simulink model "MUSIC_repo_DA_I"  (R2016a)
settings: Solver=VariableStepAuto  StartTime=0.0  StopTime=20000  RelTol=1e-3
undefined symbols (not defined in the file): S_V
libraries: xbsIndex_r4 x785, hdlsllib x7, dspbuff3 x7, dspswit3 x1
(part 1 of 8)
settings Model: Creator=Test  LastModifiedBy=Home

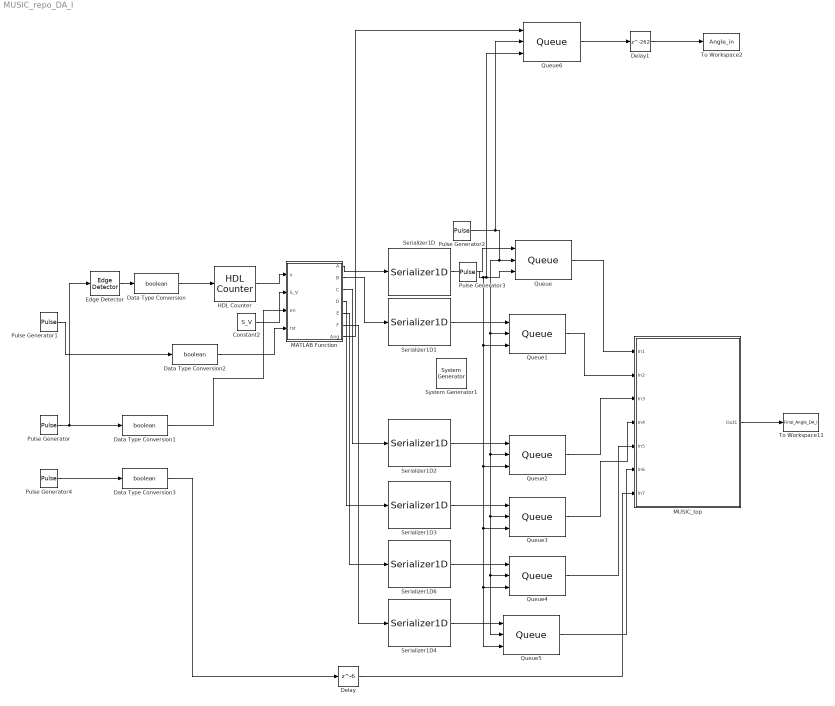
== system MUSIC_repo_DA_I ==
  " System Generator1" : xbsIndex_r4/ System Generator  Tag=genX  xilinxfamily=zynq  part=xc7z020  speed=-1  package=clg484  synthesis_tool=Vivado  clock_wrapper=Clock Enables  directory=C:/Users/Home/Desktop/Patent/Response_to_reviews_25_Feb/MUSIC_nopt  proj_type=Vivado  Synth_file=Vivado Synthesis Defaults  Impl_file=Vivado Implementation Defaults  testbench=on  simulink_period=1  sysclk_period=10  dcm_input_clock_period=10  incr_netlist=off  trim_vbits=Everywhere in SubSystem  dbl_ovrd=According to Block Masks  core_generation=According to Block Masks  run_coregen=off  deprecated_control=off  eval_field=0  block_type=sysgen
  Constant2 : Constant  Value=S_V
  Data Type Conversion{,1..3} (4 alike) : DataTypeConversion  OutDataTypeStr=boolean
  Delay : Delay  DelayLength=6  InitialCondition=0
  Delay1 : Delay  DelayLength=262  InitialCondition=0
  Edge Detector : dspswit3/Edge Detector  InputProcessing=Columns as channels (frame based)
  HDL Counter : hdlsllib/HDL Operations/HDL Counter  CountType=Count limited  CountInit=38  CountStep=1  CountMax=94  CountFromType=Initial value  CountFrom=38  CountResetPort=off  CountLoadPort=off  CountEnbPort=on  CountDirPort=off  CountDataType=Unsigned  CountWordLen=8  CountFracLen=0  CountSampTime=1
  MATLAB Function : MATLAB Function  TreatAsAtomicUnit=on
  MUSIC_top : Subsystem
  Pulse Generator : DiscretePulseGenerator  Period=90  PulseWidth=4  PhaseDelay=2
  Pulse Generator1 : DiscretePulseGenerator  Period=360
  Pulse Generator2 : DiscretePulseGenerator  PulseType=Time based  Period=0.25  PulseWidth=50
  Pulse Generator3 : DiscretePulseGenerator  PulseType=Time based  Period=1  PulseWidth=50
  Pulse Generator4 : DiscretePulseGenerator  Period=352  PulseWidth=4  PhaseDelay=2
  Queue{,1..6} (7 alike) : dspbuff3/Queue  depth=8  trigger=Rising edge  overflow=Dynamic reallocation  pes=Warning  eso=off  fso=off  nso=off  clr=off  clrOutport=off  adf=on
  Serializer1D{,1..4,6} (6 alike) : hdlsllib/HDL Operations/Serializer1D  Ratio=4  IdleCycles=0  validIn=off  startOut=off  validOut=off  inputDataDimensions=-1  inputSampleTime=-1  inputSignalType=auto
  To Workspace11 : ToWorkspace  VariableName=Final_Angle_DA_I  SampleTime=-1
  To Workspace2 : ToWorkspace  VariableName=Angle_in  SampleTime=-1
  wires:
  Data Type Conversion/1 -> HDL Counter/1
  Constant2/1 -> MATLAB Function/2(S_V)
  HDL Counter/1 -> MATLAB Function/1(x)
  Edge Detector/1 -> Data Type Conversion/1
  Pulse Generator1/1 -> Data Type Conversion2/1
  Data Type Conversion2/1 -> MATLAB Function/4(rst)
  Data Type Conversion1/1 -> MATLAB Function/3(en)
  Pulse Generator/1 -> Edge Detector/1, Data Type Conversion1/1
  MATLAB Function/1(A) -> Serializer1D/1
  Serializer1D/1 -> Queue/1
  Pulse Generator4/1 -> Data Type Conversion3/1
  Data Type Conversion3/1 -> Delay/1
  MATLAB Function/2(B) -> Serializer1D1/1
  MATLAB Function/3(C) -> Serializer1D2/1
  MATLAB Function/4(D) -> Serializer1D3/1
  MATLAB Function/5(E) -> Serializer1D6/1
  MATLAB Function/6(F) -> Serializer1D4/1
  Serializer1D1/1 -> Queue1/1
  Serializer1D2/1 -> Queue2/1
  Serializer1D3/1 -> Queue3/1
  Serializer1D6/1 -> Queue4/1
  Serializer1D4/1 -> Queue5/1
  Queue/1 -> MUSIC_top/1(In1)
  Queue1/1 -> MUSIC_top/2(In2)
  Queue2/1 -> MUSIC_top/3(In3)
  Queue3/1 -> MUSIC_top/4(In4)
  Queue4/1 -> MUSIC_top/5(In5)
  Queue5/1 -> MUSIC_top/6(In6)
  Delay/1 -> MUSIC_top/7(In7)
  MUSIC_top/1(Out1) -> To Workspace11/1
  Pulse Generator2/1 -> Queue6/2, Queue/2, Queue2/2, Queue3/2, Queue4/2, Queue5/2, Queue1/2
  Pulse Generator3/1 -> Queue6/3, Queue/3, Queue1/3, Queue2/3, Queue3/3, Queue4/3, Queue5/3
  Queue6/1 -> Delay1/1
  MATLAB Function/7(Ang) -> Queue6/1
  Delay1/1 -> To Workspace2/1

== system MUSIC_repo_DA_I/MUSIC_top ==
  In1 : Inport
  In2 : Inport  Port=2
  In3 : Inport  Port=3
  In4 : Inport  Port=4
  In5 : Inport  Port=5
  In6 : Inport  Port=6
  In7 : Inport  Port=7
  " System Generator1" : xbsIndex_r4/ System Generator  Tag=genX  xilinxfamily=zynq  part=xc7z020  speed=-1  package=clg484  synthesis_tool=Vivado  clock_wrapper=Clock Enables  directory=./res_60  proj_type=Vivado  Synth_file=Vivado Synthesis Defaults  Impl_file=Vivado Implementation Defaults  testbench=off  simulink_period=1  sysclk_period=10  dcm_input_clock_period=10  incr_netlist=off  trim_vbits=Everywhere in SubSystem  dbl_ovrd=According to Block Masks  core_generation=According to Block Masks  run_coregen=off  deprecated_control=off  eval_field=0  block_type=sysgen
  A : xbsIndex_r4/Gateway In  gui_display_data_type=Fixed-point  arith_type=Unsigned  n_bits=14  bin_pt=0  preci_type=Single  exp_width=8  frac_width=24  rows=1  columns=1  quantization="Round  (unbiased: +/- Inf)"  overflow=Saturate  period=1  UseAsADC=off  ADCChannel='1'  interface=None  automatic_assignment=on  address_offset=hex2dec('00')  intf_name=''  intf_description=''  default_value=0  timing_constraint=None  locs_specified=off  LOCs={}  io_standard={}  inherit_from_input=off  hdl_port=on  dbl_ovrd=off  block_type=gatewayin
  B : xbsIndex_r4/Gateway In  gui_display_data_type=Fixed-point  arith_type=Unsigned  n_bits=14  bin_pt=0  preci_type=Single  exp_width=8  frac_width=24  rows=1  columns=1  quantization="Round  (unbiased: +/- Inf)"  overflow=Saturate  period=1  UseAsADC=off  ADCChannel='1'  interface=None  automatic_assignment=on  address_offset=hex2dec('00')  intf_name=''  intf_description=''  default_value=0  timing_constraint=None  locs_specified=off  LOCs={}  io_standard={}  inherit_from_input=off  hdl_port=on  dbl_ovrd=off  block_type=gatewayin
  C : xbsIndex_r4/Gateway In  gui_display_data_type=Fixed-point  arith_type=Unsigned  n_bits=14  bin_pt=0  preci_type=Single  exp_width=8  frac_width=24  rows=1  columns=1  quantization="Round  (unbiased: +/- Inf)"  overflow=Saturate  period=1  UseAsADC=off  ADCChannel='1'  interface=None  automatic_assignment=on  address_offset=hex2dec('00')  intf_name=''  intf_description=''  default_value=0  timing_constraint=None  locs_specified=off  LOCs={}  io_standard={}  inherit_from_input=off  hdl_port=on  dbl_ovrd=off  block_type=gatewayin
  D : xbsIndex_r4/Gateway In  gui_display_data_type=Fixed-point  arith_type=Unsigned  n_bits=14  bin_pt=0  preci_type=Single  exp_width=8  frac_width=24  rows=1  columns=1  quantization="Round  (unbiased: +/- Inf)"  overflow=Saturate  period=1  UseAsADC=off  ADCChannel='1'  interface=None  automatic_assignment=on  address_offset=hex2dec('00')  intf_name=''  intf_description=''  default_value=0  timing_constraint=None  locs_specified=off  LOCs={}  io_standard={}  inherit_from_input=off  hdl_port=on  dbl_ovrd=off  block_type=gatewayin
  E : xbsIndex_r4/Gateway In  gui_display_data_type=Fixed-point  arith_type=Unsigned  n_bits=14  bin_pt=0  preci_type=Single  exp_width=8  frac_width=24  rows=1  columns=1  quantization="Round  (unbiased: +/- Inf)"  overflow=Saturate  period=1  UseAsADC=off  ADCChannel='1'  interface=None  automatic_assignment=on  address_offset=hex2dec('00')  intf_name=''  intf_description=''  default_value=0  timing_constraint=None  locs_specified=off  LOCs={}  io_standard={}  inherit_from_input=off  hdl_port=on  dbl_ovrd=off  block_type=gatewayin
  Enable : xbsIndex_r4/Gateway In  gui_display_data_type=Boolean  arith_type=Boolean  n_bits=14  bin_pt=0  preci_type=Single  exp_width=8  frac_width=24  rows=1  columns=1  quantization="Round  (unbiased: +/- Inf)"  overflow=Saturate  period=1  UseAsADC=off  ADCChannel='1'  interface=None  automatic_assignment=on  address_offset=hex2dec('00')  intf_name=''  intf_description=''  default_value=0  timing_constraint=None  locs_specified=off  LOCs={}  io_standard={}  inherit_from_input=off  hdl_port=on  dbl_ovrd=off  block_type=gatewayin
  F : xbsIndex_r4/Gateway In  gui_display_data_type=Fixed-point  arith_type=Unsigned  n_bits=14  bin_pt=0  preci_type=Single  exp_width=8  frac_width=24  rows=1  columns=1  quantization="Round  (unbiased: +/- Inf)"  overflow=Saturate  period=1  UseAsADC=off  ADCChannel='1'  interface=None  automatic_assignment=on  address_offset=hex2dec('00')  intf_name=''  intf_description=''  default_value=0  timing_constraint=None  locs_specified=off  LOCs={}  io_standard={}  inherit_from_input=off  hdl_port=on  dbl_ovrd=off  block_type=gatewayin
  Final_Angle_DA_I : xbsIndex_r4/Gateway Out  inherit_from_input=off  hdl_port=on  rows=1  columns=1  UseAsDAC=off  DACChannel='1'  interface=None  automatic_assignment=on  address_offset=hex2dec('00')  intf_name=''  intf_description=''  timing_constraint=None  locs_specified=off  LOCs={}  io_standard={}  block_type=gatewayout
  MUSIC : Subsystem
  Out1 : Outport
  wires:
  A/1 -> MUSIC/1(A)
  B/1 -> MUSIC/2(B)
  C/1 -> MUSIC/3(C)
  E/1 -> MUSIC/5(E)
  Enable/1 -> MUSIC/7(EN)
  MUSIC/1(Angle) -> Final_Angle_DA_I/1
  F/1 -> MUSIC/6(F)
  D/1 -> MUSIC/4(D)
  In7/1 -> Enable/1
  In1/1 -> A/1
  In2/1 -> B/1
  In4/1 -> D/1
  In3/1 -> C/1
  In6/1 -> F/1
  In5/1 -> E/1
  Final_Angle_DA_I/1 -> Out1/1

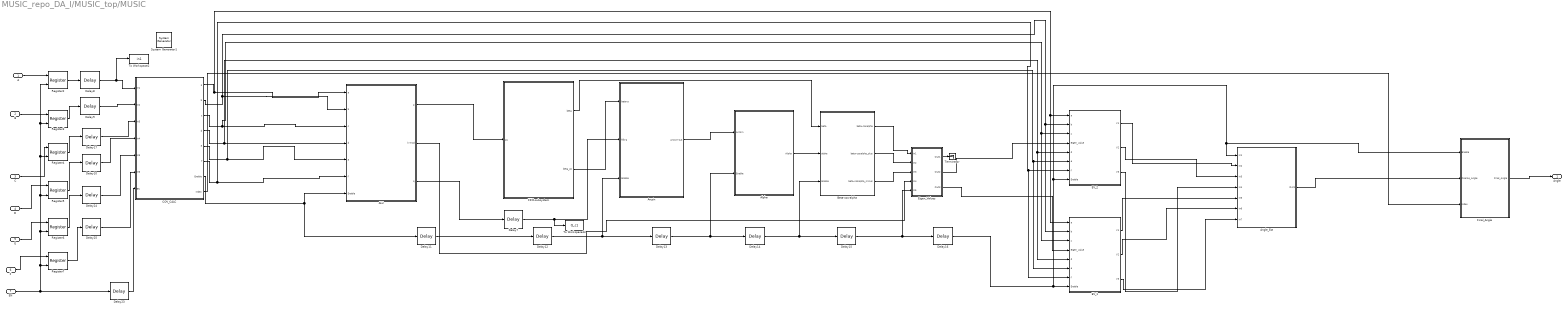
== system MUSIC_repo_DA_I/MUSIC_top/MUSIC ==
  A : Inport
  B : Inport  Port=2
  C : Inport  Port=3
  D : Inport  Port=4
  E : Inport  Port=5
  F : Inport  Port=6
  EN : Inport  Port=7
  " System Generator1" : xbsIndex_r4/ System Generator  Tag=genX  xilinxfamily=zynq  part=xc7z020  speed=-1  package=clg484  synthesis_tool=Vivado  clock_wrapper=Clock Enables  directory=./res_60  proj_type=Vivado  Synth_file=Vivado Synthesis Defaults  Impl_file=Vivado Implementation Defaults  testbench=off  simulink_period=1  sysclk_period=10  dcm_input_clock_period=10  incr_netlist=off  trim_vbits=Everywhere in SubSystem  dbl_ovrd=According to Block Masks  core_generation=According to Block Masks  run_coregen=off  deprecated_control=off  eval_field=0  block_type=sysgen
  ALU : Subsystem
  Alpha : Subsystem
  "Angle_Est " : Subsystem
  Arcsin : Subsystem
  Beta-cos-alpha : Subsystem
  COV_CALC : Subsystem
  Delay{8..10,17,23..25} (7 alike) : xbsIndex_r4/Delay  rst=off  infoeditControl=Selection of Reset will increase slice count due to use of real FFs and instead of SRLs  en=off  latency=9  reg_retiming=off  dbl_ovrd=off  block_type=delay
  Delay11 : xbsIndex_r4/Delay  rst=off  infoeditControl=Selection of Reset will increase slice count due to use of real FFs and instead of SRLs  en=off  latency=15  reg_retiming=off  dbl_ovrd=off  block_type=delay
  Delay12 : xbsIndex_r4/Delay  rst=off  infoeditControl=Selection of Reset will increase slice count due to use of real FFs and instead of SRLs  en=off  latency=10  reg_retiming=off  dbl_ovrd=off  block_type=delay
  Delay13 : xbsIndex_r4/Delay  rst=off  infoeditControl=Selection of Reset will increase slice count due to use of real FFs and instead of SRLs  en=off  latency=56  reg_retiming=off  dbl_ovrd=off  block_type=delay
  Delay14 : xbsIndex_r4/Delay  rst=off  infoeditControl=Selection of Reset will increase slice count due to use of real FFs and instead of SRLs  en=off  latency=2  reg_retiming=off  dbl_ovrd=off  block_type=delay
  Delay15 : xbsIndex_r4/Delay  rst=off  infoeditControl=Selection of Reset will increase slice count due to use of real FFs and instead of SRLs  en=off  latency=13  reg_retiming=off  dbl_ovrd=off  block_type=delay
  Delay16 : xbsIndex_r4/Delay  rst=off  infoeditControl=Selection of Reset will increase slice count due to use of real FFs and instead of SRLs  en=off  latency=1  reg_retiming=off  dbl_ovrd=off  block_type=delay
  Delay7 : xbsIndex_r4/Delay  rst=off  infoeditControl=Selection of Reset will increase slice count due to use of real FFs and instead of SRLs  en=off  latency=11  reg_retiming=off  dbl_ovrd=off  block_type=delay
  EV_1 : Subsystem
  EV_2 : Subsystem
  Eigen_Values : Subsystem
  FIFO-subsystem : Subsystem
  Final_Angle : Subsystem
  Register{2..7} (6 alike) : xbsIndex_r4/Register  init=0  rst=off  en=on  dbl_ovrd=off  block_type=register
  Terminator : Terminator
  To Workspace2 : ToWorkspace  VariableName=in1  SaveFormat=Timeseries  SampleTime=-1
  To Workspace43 : ToWorkspace  VariableName=Q_c1  SaveFormat=Timeseries  SampleTime=-1
  Angle : Outport
  wires:
  Delay13/1 -> Alpha/2(Enable), Delay14/1
  Delay14/1 -> Beta-cos-alpha/3(Enable), Delay15/1
  FIFO-subsystem/1(beta) -> Beta-cos-alpha/1(beta)
  Delay15/1 -> Eigen_Values/5(In5), Delay16/1
  Delay12/1 -> Arcsin/3(Enable), Delay13/1
  ALU/1(p) -> FIFO-subsystem/1(p1)
  Delay11/1 -> Delay12/1
  EV_2/3(V3) -> "Angle_Est "/4(In4)
  EV_1/3(V3) -> "Angle_Est "/7(In7)
  A/1 -> Register2/1
  Delay16/1 -> EV_1/8(Enable), EV_2/8(Enable), Final_Angle/1(Enable), "Angle_Est "/1(In1)
  EV_2/1(V1) -> "Angle_Est "/2(In2)
  EV_2/2(V2) -> "Angle_Est "/3(In3)
  EN/1 -> Register7/2, Register6/2, Register5/2, Register3/2, Register2/2, Register4/2, Delay23/1
  EV_1/2(V2) -> "Angle_Est "/6(In6)
  EV_1/1(V1) -> "Angle_Est "/5(In5)
  Register2/1 -> Delay8/1
  COV_CALC/2(b) -> EV_2/2(b), EV_1/2(b), ALU/2(b)
  Register6/1 -> Delay24/1
  COV_CALC/3(c) -> ALU/3(c), EV_2/3(c), EV_1/3(c)
  D/1 -> Register5/1
  C/1 -> Register4/1
  E/1 -> Register6/1
  F/1 -> Register7/1
  Register5/1 -> Delay10/1
  FIFO-subsystem/2(beta_pc) -> Arcsin/1(beta-p)
  Register3/1 -> Delay9/1
  Register7/1 -> Delay25/1
  COV_CALC/1(a) -> EV_2/1(a), EV_1/1(a), ALU/1(a)
  B/1 -> Register3/1
  Register4/1 -> Delay17/1
  Delay8/1 -> To Workspace2/1, COV_CALC/1(In1)
  "Angle_Est "/1(Out1) -> Final_Angle/2(Coarse_Angle)
  COV_CALC/7(Enable) -> Delay11/1, ALU/7(Enable)
  Delay7/1 -> Arcsin/2(fifo-q), To Workspace43/1
  COV_CALC/4(d) -> EV_2/5(d), EV_1/5(d), ALU/4(d)
  COV_CALC/6(f) -> ALU/6(f), EV_2/7(f), EV_1/7(f)
  Final_Angle/1(Final_Angle) -> Angle/1
  Delay10/1 -> COV_CALC/4(In4)
  ALU/2(k-mod) -> Eigen_Values/4(In4)
  Delay17/1 -> COV_CALC/3(In3)
  Delay24/1 -> COV_CALC/5(In5)
  COV_CALC/5(e) -> EV_2/6(e), EV_1/6(e), ALU/5(e)
  Delay9/1 -> COV_CALC/2(In2)
  Delay25/1 -> COV_CALC/6(In6)
  COV_CALC/8(Index) -> Final_Angle/3(Index)
  Delay23/1 -> COV_CALC/7(EN)
  Arcsin/1(Arcsin-out) -> Alpha/1(Arcsin)
  ALU/3(q) -> Delay7/1
  Alpha/1(Alpha) -> Beta-cos-alpha/2(alpha)
  Beta-cos-alpha/1(beta-cosalpha) -> Eigen_Values/1(In1)
  Beta-cos-alpha/2(beta-cosalpha_plus) -> Eigen_Values/2(In2)
  Beta-cos-alpha/3(beta-cosalpha_minus) -> Eigen_Values/3(In3)
  Eigen_Values/3(Out3) -> EV_1/4(Eigen_value)
  Eigen_Values/2(Out2) -> EV_2/4(Eigen_value)
  Eigen_Values/1(Out1) -> Terminator/1

== system MUSIC_repo_DA_I/MUSIC_top/MUSIC/ALU ==
  a : Inport
  b : Inport  Port=2
  c : Inport  Port=3
  d : Inport  Port=4
  e : Inport  Port=5
  f : Inport  Port=6
  Enable : Inport  Port=7
  " System Generator1" : xbsIndex_r4/ System Generator  Tag=genX  xilinxfamily=zynq  part=xc7z020  speed=-1  package=clg484  synthesis_tool=Vivado  clock_wrapper=Clock Enables  directory=./res_60  proj_type=Vivado  Synth_file=Vivado Synthesis Defaults  Impl_file=Vivado Implementation Defaults  testbench=off  simulink_period=1  sysclk_period=10  dcm_input_clock_period=10  incr_netlist=off  trim_vbits=Everywhere in SubSystem  dbl_ovrd=According to Block Masks  core_generation=According to Block Masks  run_coregen=off  deprecated_control=off  eval_field=0  block_type=sysgen
  Delay11 : xbsIndex_r4/Delay  rst=off  infoeditControl=Selection of Reset will increase slice count due to use of real FFs and instead of SRLs  en=off  latency=6  reg_retiming=off  dbl_ovrd=off  block_type=delay
  KLM-Module : Subsystem
  Module-p : Subsystem
  Module-q : Subsystem
  p : Outport
  k-mod : Outport  Port=2
  q : Outport  Port=3
  wires:
  Module-p/1(p) -> p/1
  KLM-Module/4(m) -> Module-q/2(m)
  Delay11/1 -> Module-q/5(Enable), Module-p/3(Enable)
  KLM-Module/3(l) -> Module-q/3(l), Module-p/2(l)
  KLM-Module/2(k_mod) -> k-mod/1
  Module-p/2(k^2) -> Module-q/4(k^2)
  KLM-Module/1(k) -> Module-q/1(k), Module-p/1(k)
  Module-q/1(q) -> q/1
  Enable/1 -> KLM-Module/7(Enable), Delay11/1
  e/1 -> KLM-Module/5(e)
  c/1 -> KLM-Module/3(c)
  b/1 -> KLM-Module/2(b)
  d/1 -> KLM-Module/4(d)
  f/1 -> KLM-Module/6(f)
  a/1 -> KLM-Module/1(a)

== system MUSIC_repo_DA_I/MUSIC_top/MUSIC/Alpha ==
  Arcsin : Inport
  Enable : Inport  Port=2
  " System Generator1" : xbsIndex_r4/ System Generator  Tag=genX  xilinxfamily=zynq  part=xc7z020  speed=-1  package=clg484  synthesis_tool=Vivado  clock_wrapper=Clock Enables  directory=./res_60  proj_type=Vivado  Synth_file=Vivado Synthesis Defaults  Impl_file=Vivado Implementation Defaults  testbench=off  simulink_period=1  sysclk_period=10  dcm_input_clock_period=10  incr_netlist=off  trim_vbits=Everywhere in SubSystem  dbl_ovrd=According to Block Masks  core_generation=According to Block Masks  run_coregen=off  deprecated_control=off  eval_field=0  block_type=sysgen
  AddSub3 : xbsIndex_r4/AddSub  mode=Subtraction  use_carryin=off  use_carryout=off  en=on  latency=1  precision=User Defined  arith_type="Signed  (2's comp)"  n_bits=9  bin_pt=8  quantization=Truncate  overflow=Wrap  use_behavioral_HDL=off  hw_selection=Fabric  pipelined=off  dbl_ovrd=off  block_type=addsub
  CMult1 : xbsIndex_r4/CMult  const=0.333  gui_display_data_type=Fixed-point  const_n_bits=7  const_bin_pt=6  float_type=Single  exp_bits=8  fraction_bits=24  en=off  latency=1  precision=User Defined  arith_type="Signed  (2's comp)"  n_bits=9  bin_pt=8  quantization=Truncate  overflow=Wrap  use_behavioral_HDL=off  mem_type=Distributed RAM  pipeline=off  dbl_ovrd=off  block_type=cmult
  pi/2 : xbsIndex_r4/Constant  const=1.5708  gui_display_data_type=Fixed-point  arith_type=Unsigned  n_bits=14  bin_pt=12  preci_type=Single  exp_width=8  frac_width=24  explicit_period=on  period=1  equ=P=C  opselect=C  inp2=PCIN>>17  opr=+  inp1=P  carry=CIN  dbl_ovrd=off  block_type=constant
  Alpha : Outport
  wires:
  CMult1/1 -> Alpha/1
  AddSub3/1 -> CMult1/1
  pi/2/1 -> AddSub3/1
  Arcsin/1 -> AddSub3/2
  Enable/1 -> AddSub3/3

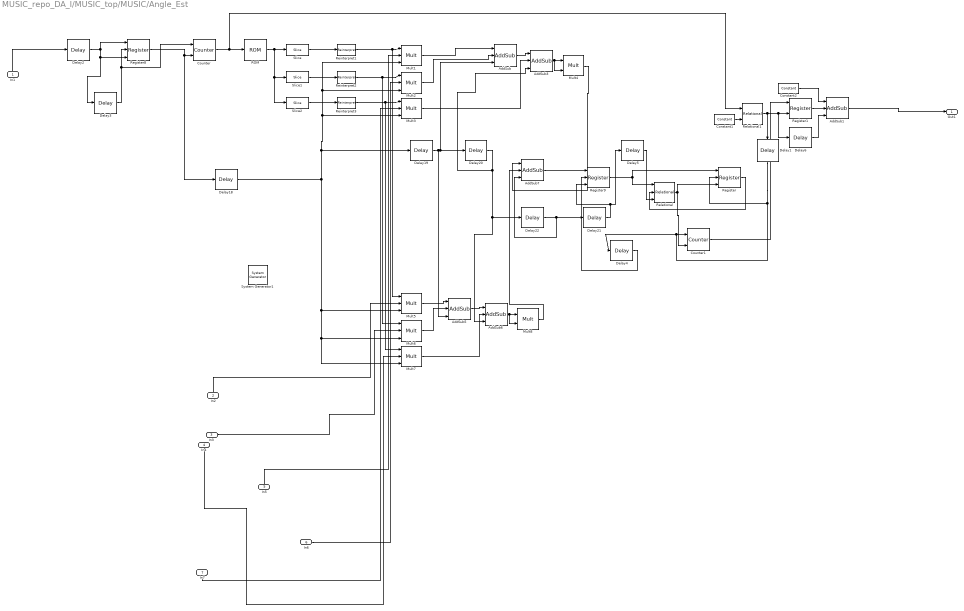
== system MUSIC_repo_DA_I/MUSIC_top/MUSIC/Angle_Est  ==
  In1 : Inport
  In2 : Inport  Port=2
  In3 : Inport  Port=3
  In4 : Inport  Port=4
  In5 : Inport  Port=5
  In6 : Inport  Port=6
  In7 : Inport  Port=7
  " System Generator1" : xbsIndex_r4/ System Generator  Tag=genX  xilinxfamily=zynq  part=xc7z020  speed=-1  package=clg484  synthesis_tool=Vivado  clock_wrapper=Clock Enables  directory=./res_60  proj_type=Vivado  Synth_file=Vivado Synthesis Defaults  Impl_file=Vivado Implementation Defaults  testbench=off  simulink_period=1  sysclk_period=10  dcm_input_clock_period=10  incr_netlist=off  trim_vbits=Everywhere in SubSystem  dbl_ovrd=According to Block Masks  core_generation=According to Block Masks  run_coregen=off  deprecated_control=off  eval_field=0  block_type=sysgen
  AddSub{,3,5..7} (5 alike) : xbsIndex_r4/AddSub  mode=Addition  use_carryin=off  use_carryout=off  en=on  latency=1  precision=User Defined  arith_type="Signed  (2's comp)"  n_bits=15  bin_pt=12  quantization=Truncate  overflow=Wrap  use_behavioral_HDL=off  hw_selection=Fabric  pipelined=off  dbl_ovrd=off  block_type=addsub
  AddSub1 : xbsIndex_r4/AddSub  mode=Addition  use_carryin=off  use_carryout=off  en=on  latency=1  precision=User Defined  arith_type=Unsigned  n_bits=8  bin_pt=0  quantization=Truncate  overflow=Wrap  use_behavioral_HDL=off  hw_selection=Fabric  pipelined=off  dbl_ovrd=off  block_type=addsub
  Constant1 : xbsIndex_r4/Constant  const=65  gui_display_data_type=Fixed-point  arith_type=Unsigned  n_bits=7  bin_pt=0  preci_type=Single  exp_width=8  frac_width=24  explicit_period=on  period=1  equ=P=C  opselect=C  inp2=PCIN>>17  opr=+  inp1=P  carry=CIN  dbl_ovrd=off  block_type=constant
  Constant2 : xbsIndex_r4/Constant  const=35  gui_display_data_type=Fixed-point  arith_type=Unsigned  n_bits=7  bin_pt=0  preci_type=Single  exp_width=8  frac_width=24  explicit_period=on  period=1  equ=P=C  opselect=C  inp2=PCIN>>17  opr=+  inp1=P  carry=CIN  dbl_ovrd=off  block_type=constant
  Counter : xbsIndex_r4/Counter  cnt_type=Count Limited  cnt_to=69  operation=Up  start_count=0  cnt_by_val=1  arith_type=Unsigned  n_bits=7  bin_pt=0  load_pin=off  rst=on  en=on  explicit_period=on  period=1  use_behavioral_HDL=off  implementation=Fabric  dbl_ovrd=off  block_type=counter
  Counter1 : xbsIndex_r4/Counter  cnt_type=Count Limited  cnt_to=70  operation=Up  start_count=0  cnt_by_val=1  arith_type=Unsigned  n_bits=8  bin_pt=0  load_pin=off  rst=on  en=on  explicit_period=on  period=1  use_behavioral_HDL=off  implementation=Fabric  dbl_ovrd=off  block_type=counter
  Delay1 : xbsIndex_r4/Delay  rst=off  infoeditControl=Selection of Reset will increase slice count due to use of real FFs and instead of SRLs  en=off  latency=10  reg_retiming=off  dbl_ovrd=off  block_type=delay
  Delay{5..6,18,20..22} (6 alike) : xbsIndex_r4/Delay  rst=off  infoeditControl=Selection of Reset will increase slice count due to use of real FFs and instead of SRLs  en=off  latency=1  reg_retiming=off  dbl_ovrd=off  block_type=delay
  Delay19 : xbsIndex_r4/Delay  rst=off  infoeditControl=Selection of Reset will increase slice count due to use of real FFs and instead of SRLs  en=off  latency=2  reg_retiming=off  dbl_ovrd=off  block_type=delay
  Delay2 : xbsIndex_r4/Delay  rst=off  infoeditControl=Selection of Reset will increase slice count due to use of real FFs and instead of SRLs  en=off  latency=43  reg_retiming=off  dbl_ovrd=off  block_type=delay
  Delay3 : xbsIndex_r4/Delay  rst=off  infoeditControl=Selection of Reset will increase slice count due to use of real FFs and instead of SRLs  en=off  latency=66  reg_retiming=off  dbl_ovrd=off  block_type=delay
  Delay4 : xbsIndex_r4/Delay  rst=off  infoeditControl=Selection of Reset will increase slice count due to use of real FFs and instead of SRLs  en=off  latency=10  reg_retiming=off  dbl_ovrd=off  block_type=delay
  Mult{1..3,5..7} (6 alike) : xbsIndex_r4/Mult  precision=User Defined  arith_type="Signed  (2's comp)"  n_bits=15  bin_pt=12  quantization=Truncate  overflow=Wrap  en=on  latency=1  use_behavioral_HDL=off  opt=Speed  use_embedded=on  optimum_pipeline=off  pipeline=on  dbl_ovrd=off  use_rpm=on  placement_style=Triangular  block_type=mult
  Mult4 : xbsIndex_r4/Mult  precision=User Defined  arith_type="Signed  (2's comp)"  n_bits=15  bin_pt=12  quantization=Truncate  overflow=Wrap  en=off  latency=1  use_behavioral_HDL=off  opt=Speed  use_embedded=on  optimum_pipeline=off  pipeline=on  dbl_ovrd=off  use_rpm=on  placement_style=Triangular  block_type=mult
  Mult8 : xbsIndex_r4/Mult  precision=User Defined  arith_type="Signed  (2's comp)"  n_bits=15  bin_pt=12  quantization=Truncate  overflow=Wrap  en=off  latency=1  use_behavioral_HDL=off  opt=Speed  use_embedded=on  optimum_pipeline=off  pipeline=on  dbl_ovrd=off  use_rpm=on  placement_style=Triangular  block_type=mult
  ROM : xbsIndex_r4/ROM  depth=71  initVector=ROM_less  distributed_mem=Block RAM  rst=off  init_reg=0  en=off  latency=1  gui_display_data_type=Fixed-point  arith_type=Unsigned  n_bits=36  bin_pt=0  preci_type=Single  exp_width=8  frac_width=24  optimize=Speed  use_rpm=on  dbl_ovrd=off  block_type=sprom
  Register : xbsIndex_r4/Register  init=1  rst=on  en=on  dbl_ovrd=off  block_type=register
  Register1 : xbsIndex_r4/Register  init=1  rst=off  en=on  dbl_ovrd=off  block_type=register
  Register8 : xbsIndex_r4/Register  init=0  rst=on  en=on  dbl_ovrd=off  block_type=register
  Register9 : xbsIndex_r4/Register  init=0  rst=on  en=on  dbl_ovrd=off  block_type=register
  Reinterpret1 : xbsIndex_r4/Reinterpret  force_arith_type=off  arith_type=Unsigned  force_bin_pt=on  bin_pt=12  block_type=reinterpret
  Reinterpret2 : xbsIndex_r4/Reinterpret  force_arith_type=off  arith_type=Unsigned  force_bin_pt=on  bin_pt=12  block_type=reinterpret
  Reinterpret3 : xbsIndex_r4/Reinterpret  force_arith_type=off  arith_type=Unsigned  force_bin_pt=on  bin_pt=12  block_type=reinterpret
  Relational : xbsIndex_r4/Relational  mode=a<b  op_type=Bool  en=on  latency=1  dbl_ovrd=off  block_type=relational
  Relational1 : xbsIndex_r4/Relational  mode=a=b  op_type=Bool  en=off  latency=1  dbl_ovrd=off  block_type=relational
  Slice : xbsIndex_r4/Slice  nbits=1  boolean_output=off  mode=Two Bit Locations  bit1=35  base1=LSB of Input  bit0=24  base0=LSB of Input  dbl_ovrd=off  block_type=slice
  Slice1 : xbsIndex_r4/Slice  nbits=12  boolean_output=off  mode=Two Bit Locations  bit1=23  base1=LSB of Input  bit0=12  base0=LSB of Input  dbl_ovrd=off  block_type=slice
  Slice2 : xbsIndex_r4/Slice  nbits=12  boolean_output=off  mode=Two Bit Locations  bit1=11  base1=LSB of Input  bit0=0  base0=LSB of Input  dbl_ovrd=off  block_type=slice
  Out1 : Outport
  wires:
  Slice1/1 -> Reinterpret2/1
  Mult2/1 -> AddSub/2
  ROM/1 -> Slice2/1, Slice1/1, Slice/1
  Slice/1 -> Reinterpret1/1
  Slice2/1 -> Reinterpret3/1
  AddSub/1 -> AddSub3/1
  Mult3/1 -> AddSub3/2
  AddSub3/1 -> Mult4/2, Mult4/1
  Constant1/1 -> Relational1/2
  AddSub5/1 -> AddSub6/1
  Reinterpret3/1 -> Mult7/1, Mult3/1
  AddSub6/1 -> Mult8/2, Mult8/1
  Counter1/1 -> Register1/1
  Mult5/1 -> AddSub5/1
  Mult8/1 -> AddSub7/2
  Delay22/1 -> AddSub7/3, Delay21/1
  Mult7/1 -> AddSub6/2
  Relational/1 -> Register/3, Counter1/2
  Counter/1 -> Relational1/1, ROM/1
  Mult6/1 -> AddSub5/2
  Reinterpret2/1 -> Mult6/1, Mult2/1
  Mult4/1 -> AddSub7/1
  Relational1/1 -> Delay1/1, Delay6/1, Register1/2
  Delay18/1 -> Mult3/3, Mult1/3, Mult2/3, Delay19/1, Mult6/3, Mult7/3, Mult5/3
  Register/1 -> Relational/2
  Reinterpret1/1 -> Mult5/1, Mult1/1
  Delay19/1 -> Delay20/1, AddSub/3, AddSub5/3
  Register9/1 -> Relational/1, Register/1
  Delay4/1 -> Register9/2
  Delay2/1 -> Delay3/1, Register8/3, Register8/1
  Register8/1 -> Counter/2, Delay18/1
  Mult1/1 -> AddSub/1
  Delay20/1 -> AddSub3/3, Delay22/1, AddSub6/3
  Delay21/1 -> Register9/3, Delay5/1
  Delay3/1 -> Counter/1, Register8/2
  Delay1/1 -> Register/2, Counter1/1, Delay4/1
  Delay5/1 -> Relational/3
  AddSub7/1 -> Register9/1
  In4/1 -> Mult7/2
  In2/1 -> Mult5/2
  In7/1 -> Mult3/2
  In6/1 -> Mult2/2
  In5/1 -> Mult1/2
  In1/1 -> Delay2/1
  In3/1 -> Mult6/2
  AddSub1/1 -> Out1/1
  Register1/1 -> AddSub1/2
  Constant2/1 -> AddSub1/1
  Delay6/1 -> AddSub1/3

== system MUSIC_repo_DA_I/MUSIC_top/MUSIC/Arcsin ==
  beta-p : Inport
  fifo-q : Inport  Port=2
  Enable : Inport  Port=3
  Angle for Arcsin : Subsystem
  Arcsin : Subsystem
  Delay : xbsIndex_r4/Delay  rst=off  infoeditControl=Selection of Reset will increase slice count due to use of real FFs and instead of SRLs  en=off  latency=12  reg_retiming=off  dbl_ovrd=off  block_type=delay
  Arcsin-out : Outport
  wires:
  fifo-q/1 -> Angle for Arcsin/1(q)
  beta-p/1 -> Angle for Arcsin/2(beta-p)
  Enable/1 -> Delay/1, Angle for Arcsin/3(Enable)
  Arcsin/1(Arcsin) -> Arcsin-out/1
  Delay/1 -> Arcsin/2(Enable)
  Angle for Arcsin/1(angle) -> Arcsin/1(Angle)

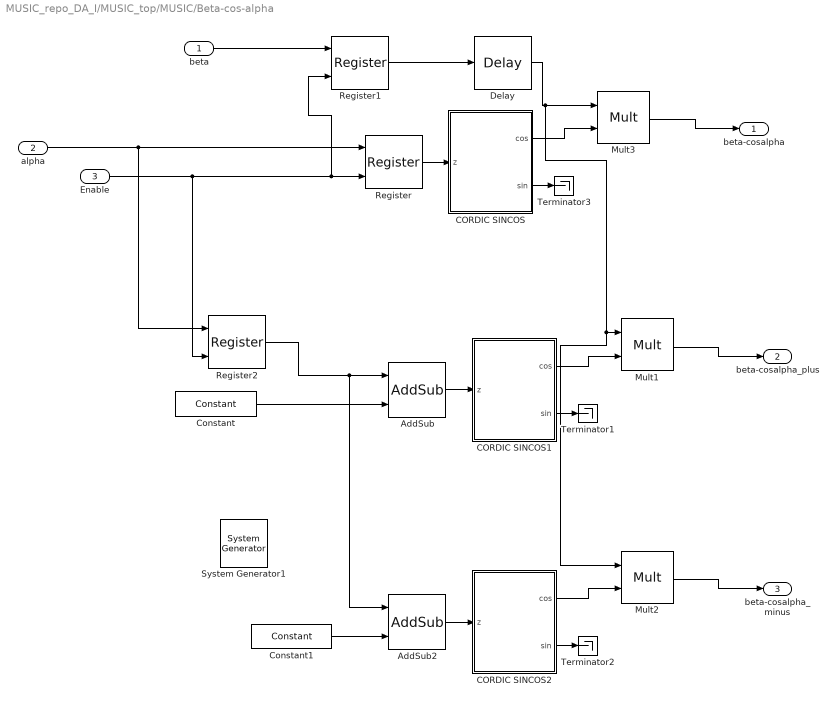
== system MUSIC_repo_DA_I/MUSIC_top/MUSIC/Beta-cos-alpha ==
  beta : Inport
  alpha : Inport  Port=2
  Enable : Inport  Port=3
  " System Generator1" : xbsIndex_r4/ System Generator  Tag=genX  xilinxfamily=zynq  part=xc7z020  speed=-1  package=clg484  synthesis_tool=Vivado  clock_wrapper=Clock Enables  directory=./res_60  proj_type=Vivado  Synth_file=Vivado Synthesis Defaults  Impl_file=Vivado Implementation Defaults  testbench=off  simulink_period=1  sysclk_period=10  dcm_input_clock_period=10  incr_netlist=off  trim_vbits=Everywhere in SubSystem  dbl_ovrd=According to Block Masks  core_generation=According to Block Masks  run_coregen=off  deprecated_control=off  eval_field=0  block_type=sysgen
  AddSub : xbsIndex_r4/AddSub  mode=Addition  use_carryin=off  use_carryout=off  en=off  latency=1  precision=User Defined  arith_type="Signed  (2's comp)"  n_bits=15  bin_pt=12  quantization=Truncate  overflow=Wrap  use_behavioral_HDL=off  hw_selection=Fabric  pipelined=off  dbl_ovrd=off  block_type=addsub
  AddSub2 : xbsIndex_r4/AddSub  mode=Subtraction  use_carryin=off  use_carryout=off  en=off  latency=1  precision=User Defined  arith_type="Signed  (2's comp)"  n_bits=15  bin_pt=12  quantization=Truncate  overflow=Wrap  use_behavioral_HDL=off  hw_selection=Fabric  pipelined=off  dbl_ovrd=off  block_type=addsub
  CORDIC SINCOS : Subsystem  mask(Xilinx CORDIC SINCOS){stages=8, pe_nbits=12, pe_binpt=8, pipeline_x=ones(1,8), prev_stages=8, pipeline=[1  1  1  1  1  1  1  1]}
      mask prompts: stages "Number of Processing Elements (integer value starting from 1)"; pe_nbits "Input Data Width"; pe_binpt "Input Binary Point Position"; pipeline_x "Latency for each Processing Element [1 0 0 1]"; prev_stages "Previous Number of Stages"; pipeline "Previous Pipeline Values"
      mask help: A parallel implementation, circular rotation mode CORDIC processor for calculating Sine and Cosine of input angle z. The number of iteration stages (and resultant output accuracy) and the processor arithmetic precision are controlled by the mask customization.
      mask init:
      | [bg,fg] = xlcmap('XBlock',0);
      | iPos = get_param(gcb,'Position');
      | iWidth=iPos(3)-iPos(1); iHeight=iPos(4)-iPos(2);
      | iCx=iWidth/2;
      | iCy=iHeight/2;
      | [logoX, logoY] = xlogo(iPos);
      | sav_gcb=gcb;
      | stages = round(sum(abs(stages)));
      | if (stages == 0)
      | 	stages = prev_stages;
      | end
      | x = zeros(1,stages);
      | pipe_size = max(size(pipeline_x));
      | if pipe_size >= stages
      | 	x(1,1:stages) = pipeline_x(1,1:stages);
      | else
      | 	x(1,1:pipe_size) = pipeline_x(1,1:pipe_size);
      | end
      | 
      | if (stages ~=prev_stages)
      | 	pipeline=x;
      | 	cordic_pe = find_system(gcb, 'lookUnderMasks', 'all', 'FollowLinks','on','masktype', 'CORDIC parallel PE');
      |     
      |   a=find_system(cordic_pe{1}, 'lookUnderMasks', 'all', 'FollowLinks','on','masktype', 'CORDIC iteration PE');
      |   for i= 2:length(a)
      |     for j=1:3
      | 	  delete_line(cordic_pe{1}, ['CORDIC PE' int2str(i-1) '/' int2str(j)], ['CORDIC PE' int2str(i) '/' int2str(j)]);
      |     end
      |   end
      |     if length(a)>0,
      |       delete_line(cordic_pe{1}, 'x/1', 'CORDIC PE1/1');
      |       delete_line(cordic_pe{1}, 'y/1', 'CORDIC PE1/2');
      |       delete_line(cordic_pe{1}, 'z/1', 'CORDIC PE1/3');
      |       delete_line(cordic_pe{1}, ['CORDIC PE' int2str(length(a)) '/1'],'X/1');
      |       delete_line(cordic_pe{1}, ['CORDIC PE' int2str(length(a)) '/2'],'Y/1');
      |       delete_line(cordic_pe{1}, ['CORDIC PE' int2str(length(a)) '/3'],'Terminator/1');
      |     elseif length(a)==0
      |       temp_port=get_param([cordic_pe{1} '/x'],'porthandles');
      |       temp_line=get_param(temp_port.Outport,'line');
      |       if temp_line>=0  delete_line(temp_line); end
      |       temp_port=get_param([cordic_pe{1} '/y'],'porthandles');
      |       temp_line=get_param(temp_port.Outport,'line');
      |       if temp_line>=0  delete_line(temp_line); end
      |       temp_port=get_param([cordic_pe{1} '/z'],'porthandles');
      |       temp_line=get_param(temp_port.Outport,'line');
      |       if temp_line>=0  delete_line(temp_line); end
      |     end
      | 
      |     for i=2:length(a)
      |       delete_block(a{i});
      |     end
      |     for i=2:stages,
      |         add_block([cordic_pe{1} '/CORDIC PE1'], [cordic_pe{1} '/CORDIC PE' int2str(i)], 'ii', int2str(i-1),'pe_nbits', 'pe_nbits','pe_binpt', 'pe_binpt','pipeline',['pipeline(1,' int2str(i) ')'],'position',[150+(i-1)*125, 70, 205+(i-1)*125, 130]);
      |     end
      | 
      |     for i= 2:stages,
      |       for j=1:3
      | 		add_line(cordic_pe{1}, ['CORDIC PE' int2str(i-1) '/' int2str(j)], ['CORDIC PE' int2str(i) '/' int2str(j)], 'autorouting', 'on');
      |       end
      |     end
      | 
      |     if stages==0
      |       add_line(cordic_pe{1}, 'x/1', 'X/1', 'autorouting', 'on');
      |       add_line(cordic_pe{1}, 'y/1', 'Terminator/1', 'autorouting', 'on');
      |       add_line(cordic_pe{1}, 'z/1', 'Z/1', 'autorouting', 'on');
      |     elseif stages>0
      |       add_line(cordic_pe{1}, 'x/1', 'CORDIC PE1/1', 'autorouting', 'on');
      |       add_line(cordic_pe{1}, 'y/1', 'CORDIC PE1/2', 'autorouting', 'on');
      |       add_line(cordic_pe{1}, 'z/1', 'CORDIC PE1/3', 'autorouting', 'on');
      | 
      |       set_param([cordic_pe{1} '/' 'X'], 'Position', [150+stages*125, 72, 180+stages*125, 86]);
      |       set_param([cordic_pe{1} '/' 'Y'], 'Position', [210+stages*125, 92, 225+stages*125, 108]);
      |       set_param([cordic_pe{1} '/' 'Terminator'], 'Position', [240+stages*125, 113, 270+stages*125, 127]);
      | 
      |       add_line(cordic_pe{1}, ['CORDIC PE' int2str(stages) '/1'], 'X/1', 'autorouting', 'on');
      |       add_line(cordic_pe{1}, ['CORDIC PE' int2str(stages) '/2'], 'Y/1', 'autorouting', 'on');
      |       add_line(cordic_pe{1}, ['CORDIC PE' int2str(stages) '/3'],'Terminator/1', 'autorouting', 'on');
      | 
      |       % force a "compile" of the constituent constant blocks to
      |       % workaround a data propagation problem
      |       find_system(cordic_pe{1}, 'lookUnderMasks', 'all', 'FollowLinks', 'on', 'MaskType','Xilinx Constant Block');
      |   end
      | 	set_param(sav_gcb, 'prev_stages', int2str(stages));
      | 	set_param(sav_gcb, 'pipeline', [ '[' int2str(x) ']']);
      | else
      | 	if (sum(pipeline~=x))
      | 		set_param(gcb, 'pipeline', [ '[' int2str(x) ']']);
      | 	end
      | end
      | str = sprintf('-%d',sum(x) + 3);
      settings: CopyFcn=set_param(gcb, 'MaskSelfModifiable', 'on', 'LinkStatus', 'none');
      mask Help: eval('');xlDoc('-book','sysgen','-topic','CORDIC_SINCOS');
      mask Display:
      | patch([0 iWidth iWidth 0],[0 0 iHeight iHeight] , bg);
      | patch(logoX,logoY , fg);
      | text(iCx-6,iCy,'z');
      | text(iCx,iCy+4,str);
      | port_label('input',1,'z');
      | port_label('output',1,'cos');
      | port_label('output',2,'sin');
      | plot([0 0 iWidth iWidth 0], [0 iHeight iHeight 0 0]);
  CORDIC SINCOS1 : Subsystem  mask(Xilinx CORDIC SINCOS){stages=8, pe_nbits=15, pe_binpt=12, pipeline_x=ones(1,8), prev_stages=8, pipeline=[1  1  1  1  1  1  1  1]}
      mask prompts: stages "Number of Processing Elements (integer value starting from 1)"; pe_nbits "Input Data Width"; pe_binpt "Input Binary Point Position"; pipeline_x "Latency for each Processing Element [1 0 0 1]"; prev_stages "Previous Number of Stages"; pipeline "Previous Pipeline Values"
      mask help: A parallel implementation, circular rotation mode CORDIC processor for calculating Sine and Cosine of input angle z. The number of iteration stages (and resultant output accuracy) and the processor arithmetic precision are controlled by the mask customization.
      mask init: same as MUSIC_repo_DA_I/MUSIC_top/MUSIC/Beta-cos-alpha/CORDIC SINCOS
      settings: CopyFcn=set_param(gcb, 'MaskSelfModifiable', 'on', 'LinkStatus', 'none');
      mask Help: eval('');xlDoc('-book','sysgen','-topic','CORDIC_SINCOS');
      mask Display:
      | patch([0 iWidth iWidth 0],[0 0 iHeight iHeight] , bg);
      | patch(logoX,logoY , fg);
      | text(iCx-6,iCy,'z');
      | text(iCx,iCy+4,str);
      | port_label('input',1,'z');
      | port_label('output',1,'cos');
      | port_label('output',2,'sin');
      | plot([0 0 iWidth iWidth 0], [0 iHeight iHeight 0 0]);
  CORDIC SINCOS2 : Subsystem  mask(Xilinx CORDIC SINCOS){stages=8, pe_nbits=15, pe_binpt=12, pipeline_x=ones(1,8), prev_stages=8, pipeline=[1  1  1  1  1  1  1  1]}
      mask prompts: stages "Number of Processing Elements (integer value starting from 1)"; pe_nbits "Input Data Width"; pe_binpt "Input Binary Point Position"; pipeline_x "Latency for each Processing Element [1 0 0 1]"; prev_stages "Previous Number of Stages"; pipeline "Previous Pipeline Values"
      mask help: A parallel implementation, circular rotation mode CORDIC processor for calculating Sine and Cosine of input angle z. The number of iteration stages (and resultant output accuracy) and the processor arithmetic precision are controlled by the mask customization.
      mask init: same as MUSIC_repo_DA_I/MUSIC_top/MUSIC/Beta-cos-alpha/CORDIC SINCOS
      settings: CopyFcn=set_param(gcb, 'MaskSelfModifiable', 'on', 'LinkStatus', 'none');
      mask Help: eval('');xlDoc('-book','sysgen','-topic','CORDIC_SINCOS');
      mask Display:
      | patch([0 iWidth iWidth 0],[0 0 iHeight iHeight] , bg);
      | patch(logoX,logoY , fg);
      | text(iCx-6,iCy,'z');
      | text(iCx,iCy+4,str);
      | port_label('input',1,'z');
      | port_label('output',1,'cos');
      | port_label('output',2,'sin');
      | plot([0 0 iWidth iWidth 0], [0 iHeight iHeight 0 0]);
  Constant : xbsIndex_r4/Constant  const=2.0944  gui_display_data_type=Fixed-point  arith_type=Unsigned  n_bits=14  bin_pt=12  preci_type=Single  exp_width=8  frac_width=24  explicit_period=on  period=1  equ=P=C  opselect=C  inp2=PCIN>>17  opr=+  inp1=P  carry=CIN  dbl_ovrd=off  block_type=constant
  Constant1 : xbsIndex_r4/Constant  const=2.0944  gui_display_data_type=Fixed-point  arith_type=Unsigned  n_bits=14  bin_pt=12  preci_type=Single  exp_width=8  frac_width=24  explicit_period=on  period=1  equ=P=C  opselect=C  inp2=PCIN>>17  opr=+  inp1=P  carry=CIN  dbl_ovrd=off  block_type=constant
  Delay : xbsIndex_r4/Delay  rst=off  infoeditControl=Selection of Reset will increase slice count due to use of real FFs and instead of SRLs  en=off  latency=11  reg_retiming=off  dbl_ovrd=off  block_type=delay
  Mult1 : xbsIndex_r4/Mult  precision=User Defined  arith_type="Signed  (2's comp)"  n_bits=16  bin_pt=12  quantization=Truncate  overflow=Wrap  en=off  latency=1  use_behavioral_HDL=off  opt=Speed  use_embedded=on  optimum_pipeline=off  pipeline=on  dbl_ovrd=off  use_rpm=on  placement_style=Triangular  block_type=mult
  Mult2 : xbsIndex_r4/Mult  precision=User Defined  arith_type="Signed  (2's comp)"  n_bits=16  bin_pt=12  quantization=Truncate  overflow=Wrap  en=off  latency=1  use_behavioral_HDL=off  opt=Speed  use_embedded=on  optimum_pipeline=off  pipeline=on  dbl_ovrd=off  use_rpm=on  placement_style=Triangular  block_type=mult
  Mult3 : xbsIndex_r4/Mult  precision=Full  arith_type="Signed  (2's comp)"  n_bits=9  bin_pt=8  quantization=Truncate  overflow=Wrap  en=off  latency=1  use_behavioral_HDL=off  opt=Speed  use_embedded=on  optimum_pipeline=off  pipeline=on  dbl_ovrd=off  use_rpm=on  placement_style=Triangular  block_type=mult
  Register : xbsIndex_r4/Register  init=0  rst=off  en=on  dbl_ovrd=off  block_type=register
  Register1 : xbsIndex_r4/Register  init=0  rst=off  en=on  dbl_ovrd=off  block_type=register
  Register2 : xbsIndex_r4/Register  init=0  rst=off  en=on  dbl_ovrd=off  block_type=register
  Terminator1 : Terminator
  Terminator2 : Terminator
  Terminator3 : Terminator
  beta-cosalpha : Outport
  beta-cosalpha_plus : Outport  Port=2
  beta-cosalpha_minus : Outport  Port=3
  wires:
  CORDIC SINCOS/2(sin) -> Terminator3/1
  CORDIC SINCOS/1(cos) -> Mult3/2
  Mult3/1 -> beta-cosalpha/1
  Register/1 -> CORDIC SINCOS/1(z)
  Enable/1 -> Register2/2, Register1/2, Register/2
  Register1/1 -> Delay/1
  beta/1 -> Register1/1
  CORDIC SINCOS1/2(sin) -> Terminator1/1
  CORDIC SINCOS1/1(cos) -> Mult1/2
  Mult1/1 -> beta-cosalpha_plus/1
  AddSub/1 -> CORDIC SINCOS1/1(z)
  Constant/1 -> AddSub/2
  alpha/1 -> Register2/1, Register/1
  CORDIC SINCOS2/2(sin) -> Terminator2/1
  AddSub2/1 -> CORDIC SINCOS2/1(z)
  Constant1/1 -> AddSub2/2
  Delay/1 -> Mult2/1, Mult1/1, Mult3/1
  Mult2/1 -> beta-cosalpha_minus/1
  CORDIC SINCOS2/1(cos) -> Mult2/2
  Register2/1 -> AddSub2/1, AddSub/1

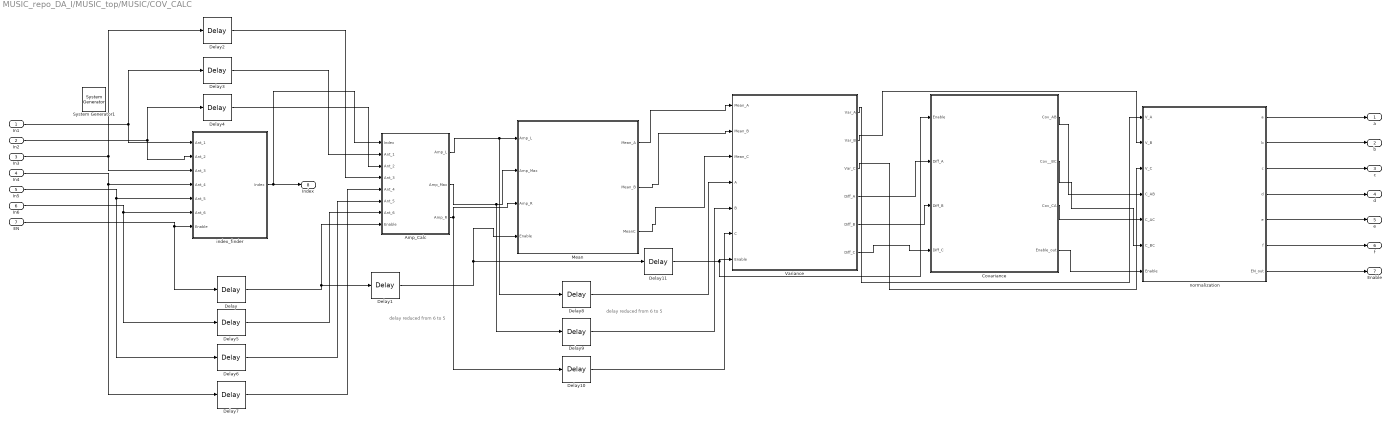
== system MUSIC_repo_DA_I/MUSIC_top/MUSIC/COV_CALC ==
  note: delay reduced from 6 to 5
  note: delay reduced from 6 to 5
  In1 : Inport
  In2 : Inport  Port=2
  In3 : Inport  Port=3
  In4 : Inport  Port=4
  In5 : Inport  Port=5
  In6 : Inport  Port=6
  EN : Inport  Port=7
  " System Generator1" : xbsIndex_r4/ System Generator  Tag=genX  xilinxfamily=zynq  part=xc7z020  speed=-1  package=clg484  synthesis_tool=Vivado  clock_wrapper=Clock Enables  directory=./res_60  proj_type=Vivado  Synth_file=Vivado Synthesis Defaults  Impl_file=Vivado Implementation Defaults  testbench=off  simulink_period=1  sysclk_period=10  dcm_input_clock_period=10  incr_netlist=off  trim_vbits=Everywhere in SubSystem  dbl_ovrd=According to Block Masks  core_generation=According to Block Masks  run_coregen=off  deprecated_control=off  eval_field=0  block_type=sysgen
  Amp_Calc : Subsystem
  Covariance : Subsystem
  Delay : xbsIndex_r4/Delay  rst=off  infoeditControl=Selection of Reset will increase slice count due to use of real FFs and instead of SRLs  en=off  latency=10  reg_retiming=off  dbl_ovrd=off  block_type=delay
  Delay1 : xbsIndex_r4/Delay  rst=off  infoeditControl=Selection of Reset will increase slice count due to use of real FFs and instead of SRLs  en=off  latency=3  reg_retiming=off  dbl_ovrd=off  block_type=delay
  Delay10 : xbsIndex_r4/Delay  rst=off  infoeditControl=Selection of Reset will increase slice count due to use of real FFs and instead of SRLs  en=off  latency=5  reg_retiming=off  dbl_ovrd=off  block_type=delay
  Delay11 : xbsIndex_r4/Delay  rst=off  infoeditControl=Selection of Reset will increase slice count due to use of real FFs and instead of SRLs  en=off  latency=2  reg_retiming=off  dbl_ovrd=off  block_type=delay
  Delay{2..7} (6 alike) : xbsIndex_r4/Delay  rst=off  infoeditControl=Selection of Reset will increase slice count due to use of real FFs and instead of SRLs  en=off  latency=9  reg_retiming=off  dbl_ovrd=off  block_type=delay
  Delay8 : xbsIndex_r4/Delay  rst=off  infoeditControl=Selection of Reset will increase slice count due to use of real FFs and instead of SRLs  en=off  latency=5  reg_retiming=off  dbl_ovrd=off  block_type=delay
  Delay9 : xbsIndex_r4/Delay  rst=off  infoeditControl=Selection of Reset will increase slice count due to use of real FFs and instead of SRLs  en=off  latency=5  reg_retiming=off  dbl_ovrd=off  block_type=delay
  Mean : Subsystem
  Variance : Subsystem
  index_finder : Subsystem
  normalization : Subsystem
  a : Outport
  b : Outport  Port=2
  c : Outport  Port=3
  d : Outport  Port=4
  e : Outport  Port=5
  f : Outport  Port=6
  Enable : Outport  Port=7
  Index : Outport  Port=8
  wires:
  In1/1 -> index_finder/1(Ant_1), Delay3/1
  In2/1 -> index_finder/2(Ant_2), Delay4/1
  In3/1 -> index_finder/3(Ant_3), Delay2/1
  In4/1 -> index_finder/4(Ant_4), Delay7/1
  In5/1 -> index_finder/5(Ant_5), Delay6/1
  In6/1 -> index_finder/6(Ant_6), Delay5/1
  EN/1 -> index_finder/7(Enable), Delay/1
  index_finder/1(Index) -> Index/1, Amp_Calc/1(Index)
  Amp_Calc/1(Amp_L) -> Delay8/1, Mean/1(Amp_L)
  Amp_Calc/2(Amp_Max) -> Delay9/1, Mean/2(Amp_Max)
  Amp_Calc/3(Amp_R) -> Delay10/1, Mean/3(Amp_R)
  Delay/1 -> Amp_Calc/8(Enable), Delay1/1
  Mean/1(Mean_A) -> Variance/1(Mean_A)
  Mean/2(Mean_B) -> Variance/2(Mean_B)
  Mean/3(MeanC) -> Variance/3(Mean_C)
  Delay2/1 -> Amp_Calc/4(Ant_3)
  Delay3/1 -> Amp_Calc/2(Ant_1)
  Delay4/1 -> Amp_Calc/3(Ant_2)
  Delay5/1 -> Amp_Calc/7(Ant_6)
  Delay6/1 -> Amp_Calc/6(Ant_5)
  Delay7/1 -> Amp_Calc/5(Ant_4)
  Delay8/1 -> Variance/4(A)
  Delay9/1 -> Variance/5(B)
  Delay10/1 -> Variance/6(C)
  Variance/1(Var_A) -> normalization/1(V_A)
  Variance/2(Var_B) -> normalization/2(V_B)
  Variance/4(Diff_A) -> Covariance/2(Diff_A)
  Variance/5(Diff_B) -> Covariance/3(Diff_B)
  Variance/6(Diff_C) -> Covariance/4(Diff_C)
  Variance/3(Var_C) -> normalization/3(V_C)
  Covariance/1(Cov_AB) -> normalization/4(C_AB)
  Covariance/2(Cov__BC) -> normalization/6(C_BC)
  Covariance/3(Cov_CA) -> normalization/5(C_AC)
  Covariance/4("Enable_out ") -> normalization/7(Enable)
  normalization/1(a) -> a/1
  normalization/2(b) -> b/1
  normalization/5(e) -> e/1
  normalization/6(f) -> f/1
  normalization/3(c) -> c/1
  normalization/4(d) -> d/1
  normalization/7(EN_out) -> Enable/1
  Delay1/1 -> Delay11/1, Mean/4(Enable)
  Delay11/1 -> Covariance/1(Enable), Variance/7(Enable)

== system MUSIC_repo_DA_I/MUSIC_top/MUSIC/EV_1 ==
  a : Inport
  b : Inport  Port=2
  c : Inport  Port=3
  Eigen_value : Inport  Port=4
  d : Inport  Port=5
  e : Inport  Port=6
  f : Inport  Port=7
  Enable : Inport  Port=8
  AddSub : xbsIndex_r4/AddSub  mode=Subtraction  use_carryin=off  use_carryout=off  en=on  latency=1  precision=User Defined  arith_type="Signed  (2's comp)"  n_bits=14  bin_pt=12  quantization=Truncate  overflow=Wrap  use_behavioral_HDL=off  hw_selection=Fabric  pipelined=off  dbl_ovrd=off  block_type=addsub
  AddSub1 : xbsIndex_r4/AddSub  mode=Subtraction  use_carryin=off  use_carryout=off  en=on  latency=1  precision=User Defined  arith_type="Signed  (2's comp)"  n_bits=14  bin_pt=12  quantization=Truncate  overflow=Wrap  use_behavioral_HDL=off  hw_selection=Fabric  pipelined=off  dbl_ovrd=off  block_type=addsub
  AddSub2 : xbsIndex_r4/AddSub  mode=Subtraction  use_carryin=off  use_carryout=off  en=on  latency=1  precision=User Defined  arith_type="Signed  (2's comp)"  n_bits=14  bin_pt=12  quantization=Truncate  overflow=Wrap  use_behavioral_HDL=off  hw_selection=Fabric  pipelined=off  dbl_ovrd=off  block_type=addsub
  Delay : xbsIndex_r4/Delay  rst=off  infoeditControl=Selection of Reset will increase slice count due to use of real FFs and instead of SRLs  en=off  latency=1  reg_retiming=off  dbl_ovrd=off  block_type=delay
  Eigen_Vector : Subsystem
  V1 : Outport
  V2 : Outport  Port=2
  V3 : Outport  Port=3
  wires:
  Eigen_Vector/1(V1) -> V1/1
  Eigen_Vector/3(V3) -> V3/1
  Enable/1 -> AddSub2/3, AddSub1/3, AddSub/3, Delay/1
  d/1 -> Eigen_Vector/5(In5)
  e/1 -> Eigen_Vector/6(In7)
  f/1 -> Eigen_Vector/7(In8)
  Eigen_Vector/2(V2) -> V2/1
  c/1 -> AddSub2/1
  AddSub1/1 -> Eigen_Vector/3(In3)
  b/1 -> AddSub1/1
  a/1 -> AddSub/1
  Delay/1 -> Eigen_Vector/1(In1)
  AddSub2/1 -> Eigen_Vector/4(In4)
  AddSub/1 -> Eigen_Vector/2(In2)
  Eigen_value/1 -> AddSub2/2, AddSub1/2, AddSub/2

== system MUSIC_repo_DA_I/MUSIC_top/MUSIC/EV_2 ==
  a : Inport
  b : Inport  Port=2
  c : Inport  Port=3
  Eigen_value : Inport  Port=4
  d : Inport  Port=5
  e : Inport  Port=6
  f : Inport  Port=7
  Enable : Inport  Port=8
  AddSub : xbsIndex_r4/AddSub  mode=Subtraction  use_carryin=off  use_carryout=off  en=on  latency=1  precision=User Defined  arith_type="Signed  (2's comp)"  n_bits=14  bin_pt=12  quantization=Truncate  overflow=Wrap  use_behavioral_HDL=off  hw_selection=Fabric  pipelined=off  dbl_ovrd=off  block_type=addsub
  AddSub1 : xbsIndex_r4/AddSub  mode=Subtraction  use_carryin=off  use_carryout=off  en=on  latency=1  precision=User Defined  arith_type="Signed  (2's comp)"  n_bits=14  bin_pt=12  quantization=Truncate  overflow=Wrap  use_behavioral_HDL=off  hw_selection=Fabric  pipelined=off  dbl_ovrd=off  block_type=addsub
  AddSub2 : xbsIndex_r4/AddSub  mode=Subtraction  use_carryin=off  use_carryout=off  en=on  latency=1  precision=User Defined  arith_type="Signed  (2's comp)"  n_bits=14  bin_pt=12  quantization=Truncate  overflow=Wrap  use_behavioral_HDL=off  hw_selection=Fabric  pipelined=off  dbl_ovrd=off  block_type=addsub
  Delay : xbsIndex_r4/Delay  rst=off  infoeditControl=Selection of Reset will increase slice count due to use of real FFs and instead of SRLs  en=off  latency=1  reg_retiming=off  dbl_ovrd=off  block_type=delay
  Eigen_Vector : Subsystem
  V1 : Outport
  V2 : Outport  Port=2
  V3 : Outport  Port=3
  wires:
  Eigen_value/1 -> AddSub/2, AddSub1/2, AddSub2/2
  AddSub/1 -> Eigen_Vector/2(In2)
  AddSub2/1 -> Eigen_Vector/4(In4)
  Delay/1 -> Eigen_Vector/1(In1)
  a/1 -> AddSub/1
  b/1 -> AddSub1/1
  AddSub1/1 -> Eigen_Vector/3(In3)
  c/1 -> AddSub2/1
  Eigen_Vector/2(V2) -> V2/1
  f/1 -> Eigen_Vector/7(In8)
  e/1 -> Eigen_Vector/6(In7)
  d/1 -> Eigen_Vector/5(In5)
  Enable/1 -> Delay/1, AddSub/3, AddSub1/3, AddSub2/3
  Eigen_Vector/3(V3) -> V3/1
  Eigen_Vector/1(V1) -> V1/1
